simulink model "Super6"  (Simulink 8.7)
settings: Solver=ode45  StartTime=0.0  StopTime=10.0  RelTol=1e-3
settings Model: Creator=scaife  LastModifiedBy=bourbouh  ExtModeAutoUpdateStatusClock=off
settings DataIOCC: SignalLoggingSaveFormat=ModelDataLogs  SignalLoggingName=sigsOut
settings DebuggingCC: SaveWithParameterizedLinksMsg=none  SignalResolutionControl=TryResolveAllWithWarning  MultiTaskDSMMsg=warning  MultiTaskCondExecSysMsg=none
settings HardwareCC: TargetUnknown=on
settings SFSimCC: SimParseCustomCode=off
settings GRTTargetCC: CombineOutputUpdateFcns=off  GRTInterface=on

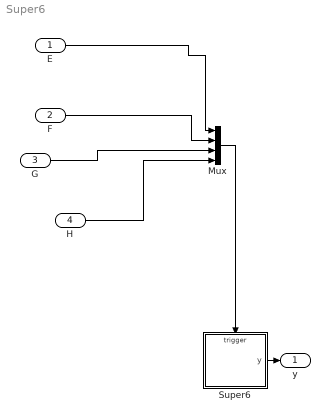
== system Super6 ==
  E : Inport
  F : Inport  Port=2
  G : Inport  Port=3
  H : Inport  Port=4
  Mux : Mux
  Super6 : Stateflow chart  TreatAsAtomicUnit=on
  y : Outport
  wires:
  Mux/1 -> Super6/Trigger
  H/1 -> Mux/4
  E/1 -> Mux/1
  F/1 -> Mux/2
  G/1 -> Mux/3
  Super6/1(y) -> y/1

== stateflow chart Super6 ==
  state A
    du: y++;
    state A1
      du:y++;
      state A1a
        du:y++;
        state A1ai
          du:y++;
        (default) -> A1ai
      (default) -> A1a
    (default) -> A1
  state B
    du:y++;
    state B1
      du:y++;
      state B1a
        du:y++;
        state B1ai
          du:y++;
        (default) -> B1ai
      (default) -> B1a
    (default) -> B1
  A -> B : E
  (default) -> A
  A1 -> B1 : F
  A1a -> B1a : G
  A1ai -> B1ai : H
  B1ai -> A1ai : H
  B1a -> A1a : G
  B1 -> A1 : F
  B -> A : E
  data: y output uint32
  events: E input EITHER_EDGE_EVENT; F input EITHER_EDGE_EVENT; G input EITHER_EDGE_EVENT; H input EITHER_EDGE_EVENT
